simulink model "buck_conv2"  (R2021a)
settings: Solver=VariableStepAuto  StartTime=0.0  StopTime=0.01  RelTol=1e-3
libraries: spsSeriesRLCBranchLib x4, spsDiodeLib x1, spsMosfetLib x1, spsMultimeterLib x1, spsPWMGeneratorDCDCLib x1, spsDCVoltageSourceLib x1, spspowerguiLib x1
settings Model: Creator=probinet  LastModifiedBy=probinet
settings SolverCC: AlgebraicLoopSolver=TrustRegion
settings DebuggingCC: SFMachineParentedDataDiag=warning

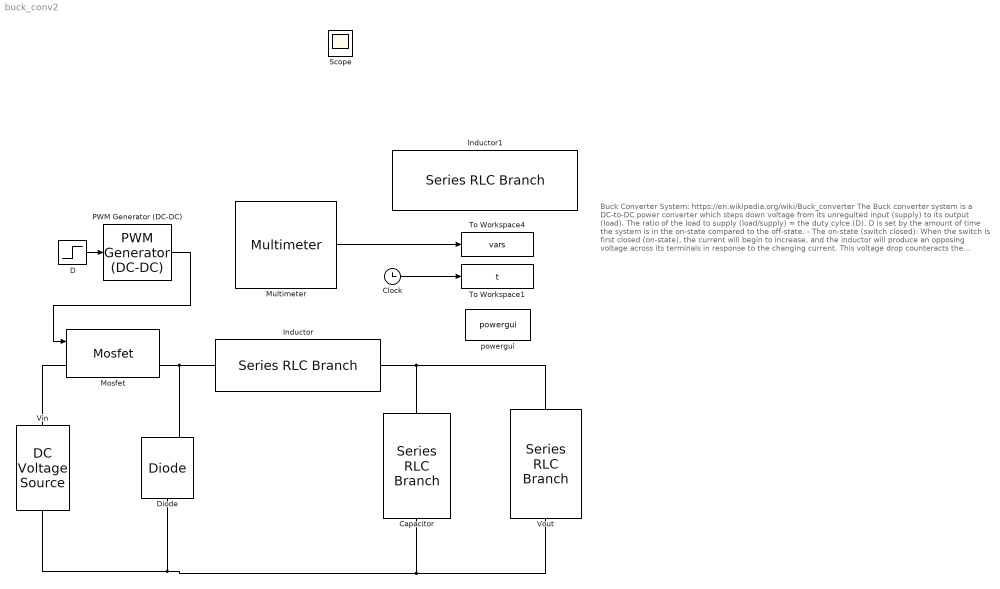
== system buck_conv2 ==
  note: Buck Converter System: https://en.wikipedia.org/wiki/Buck_converter
      | The Buck converter system is a DC-to-DC power converter which steps down voltage from its unregulted input (supply) to its output (load). The ratio of the load to supply (load/supply) = the duty cylce (D). D is set by the amount of time the system is in the on-state compared to the off-state.
      |
      | - The on-state (switch closed): When the switch is first closed (on-state), the current will begin to increase, and the inductor will produce an opposing voltage across its terminals in response to the changing current. This voltage drop counteracts the voltage of the source and therefore reduces the net voltage across the load. Over time, the rate of change of current decreases, and the voltage across the inductor also then decreases, increasing the voltage at the load.
      |
      | - The off-state (switch open): When the switch is opened again (off-state), the voltage source will be removed from the circuit, and the current will decrease. The decreasing current will produce a voltage drop across the inductor (opposite to the drop at on-state), and now the inductor becomes a current source. The stored energy in the inductor's magnetic field supports the current flow through the load. This current, flowing while the input voltage source is disconnected, when appended to the current flowing during on-state, totals to current greater than the average input current (being zero during off-state).
      |
      | Equations:
      |
      | On-state:
      | $V_L = V_i - V_o$
      | $V_L = L*(dI_L/dt)$
      | $\Delta I_L = \int_{0}^{t_o} \frac{V_L}{L} dt = \frac{V_i - V_o}{L} dt, t_o = DT$
      |
      | Off-state:
      | $V_L = -V_o$
      | $\Delta I_Loff = \int_{t_o}^{T = t_o + t_off} \frac{V_L}{L} dt = -\frac{V_o}{L}t_off, t_off = (1-D)T$
      |
      | $D = \frac{V_o}{V_i}$
  Capacitor : spsSeriesRLCBranchLib/Series RLC Branch  LConnTagsString=__new0  RConnTagsString=__new0  BranchType=C  Resistance=0.65e-3  Inductance=1e-3  SetiL0=off  InitialCurrent=0  Capacitance=30e-6  Setx0=off  InitialVoltage=0  Measurements=None
  Clock : Clock
  D : Step  Time=0.005  Before=0.2  After=0.5  SampleTime=0
  Diode : spsDiodeLib/Diode  Ron=0.001  Lon=0  Vf=0.8  IC=0  UseSnubber=0  Rs=500  Cs=250e-9  Measurements=on
  Inductor : spsSeriesRLCBranchLib/Series RLC Branch  LConnTagsString=__new0  RConnTagsString=__new0  BranchType=L  Resistance=0.02  Inductance=3e-3  SetiL0=off  InitialCurrent=0  Capacitance=1e-6  Setx0=off  InitialVoltage=0  Measurements=Branch voltage and current
  Inductor1 : spsSeriesRLCBranchLib/Series RLC Branch  LConnTagsString=__new0  RConnTagsString=__new0  BranchType=RL  Resistance=0.02  Inductance=3e-3  SetiL0=off  InitialCurrent=0  Capacitance=1e-6  Setx0=off  InitialVoltage=0  Measurements=Branch voltage and current
  Mosfet : spsMosfetLib/Mosfet  Ron=0.1  Lon=0  Rd=0.01  Vfd=0  IC=0  Rs=1e5  Cs=inf  Measurements=on
  Multimeter : spsMultimeterLib/Multimeter  PhasorSimulation=off  OutputType=Complex  sel=[4 1 5 3 7]  L=7  Gain=[1 1 1 1 1]  yselected={'Usrc: Vin','Ub: Inductor','Ib: Inductor','Ub: Vout','Ib: Vout'};  PSBOutputType=1  PSBequivalent=0  AxesSetting=[0,0.1,-100,100]  Display=0  SavedBlockNames=-11
  PWM Generator (DC-DC) : spsPWMGeneratorDCDCLib/PWM Generator (DC-DC)  Fsw=10e3  Ts=0
  To Workspace1 : ToWorkspace  VariableName=t  SampleTime=-1
      settings: Save2DSignal=2-D array (concatenate along first dimension)
  To Workspace4 : ToWorkspace  VariableName=vars  SampleTime=-1
      settings: Save2DSignal=2-D array (concatenate along first dimension)
  Vin : spsDCVoltageSourceLib/DC Voltage Source  Amplitude=200  Measurements=Voltage
  Vout : spsSeriesRLCBranchLib/Series RLC Branch  LConnTagsString=__new0  RConnTagsString=__new0  BranchType=R  Resistance=10  Inductance=1e-3  SetiL0=off  InitialCurrent=0  Capacitance=1e-6  Setx0=off  InitialVoltage=0  Measurements=Branch voltage and current
  powergui : spspowerguiLib/powergui  Priority=1  SimulationMode=Continuous  SampleTime=50e-6  frequency=60  Iterations=50  frequencyindice=0  Pbase=100e6  ErrMax=1e-4  UnitsV=kV  UnitsW=MW  buscounter=0  FunctionMessages=off  echomessages=off  EnableUseOfTLC=off  CurrentSourceSwitches=off  DisableSnubberDevices=off  DisableRonSwitches=off  DisableVfSwitches=off  DisplayEquations=off  AutomaticDiscreteSolvers=off  SolverType=Tustin/Backward Euler (TBE)  Interpol=off  ExternalGateDelay=off  methode=off  Ts=100  x0status=blocks  SPID=on  SwTol=0  HookPort=off  NonlinearTolerance=1e-4  nMaxIteration=100  ContinueOnMaxIteration=off  RestoreLinks=warning  ResistiveCurrentMeasurement=off  Frange=[0:2:500]  Ylog=off  Xlog=on  ShowGrid=off  save=off  variable=ZData  structure=0  ZoomFFT=off  StartTime=0.0  cycles=1  DisplayStyle=1  fundamental=60  FreqAxis=off  MaxFrequency=1000  frequencyindicesteady=1  RmsSteady=1  display=off
  Scope : Scope
  wires:
  D/1 -> PWM Generator (DC-DC)/1
  PWM Generator (DC-DC)/1 -> Mosfet/1
  Clock/1 -> To Workspace1/1
  Multimeter/1 -> To Workspace4/1
  connections:
  Inductor/RConn1 -- Diode/RConn1 -- Mosfet/RConn1
  Inductor/LConn1 -- Capacitor/LConn1 -- Vout/LConn1
  Vin/LConn1 -- Diode/LConn1 -- Capacitor/RConn1 -- Vout/RConn1
  Vin/RConn1 -- Mosfet/LConn1
